simulink model "ex1"  (R2020a)
settings: Solver=VariableStepAuto  StartTime=0.0  StopTime=10.0  RelTol=1e-3

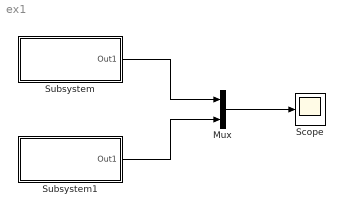
== system ex1 ==
  Mux : Mux  Inputs=2
  Scope : Scope
  Subsystem : Subsystem  mask(subsistem){a1=1, f1=2}
      mask prompts: a1 "a1="; f1 "f1="
      mask help:
      | a1 și f1 reprezintă amplitudinea respectiv frecvența
      | funcției sinus
      mask Help:
      | blocul trasează o funcție sinus de
      | amplitudine a1 și frecvență f1
      mask Callback a1:
      | if str2num(get_param(gcb,'a1'))<0
      |     error('amplitudinea este negativa')
      | end
      mask Callback f1:
      | if str2num(get_param(gcb,'f1'))<0
      |     error('frecventa este negativa')
      | end
  Subsystem1 : Subsystem  mask(subsitem){a2=1, f2=3}
      mask prompts: a2 "a2="; f2 "f2="
      mask help:
      | a1 și f1 reprezintă amplitudinea respectiv frecvența
      | funcției sinus
      mask Help:
      | blocul trasează o funcție sinus de
      | amplitudine a1 și frecvență f1
      mask Callback a2:
      | if str2num(get_param(gcb,'a2'))<0
      |     error('Amplitudinea este negativa!')
      | end
      mask Callback f2:
      | if str2num(get_param(gcb,'f2'))<0
      |     error('Amplitudinea este negativa!')
      | end
  wires:
  Subsystem/1(Out1) -> Mux/1
  Subsystem1/1(Out1) -> Mux/2
  Mux/1 -> Scope/1

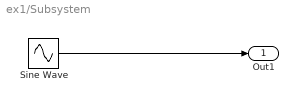
== system ex1/Subsystem ==
  Sine Wave : Sin  Amplitude=a1  Frequency=f1  SampleTime=0
  Out1 : Outport
  wires:
  Sine Wave/1 -> Out1/1

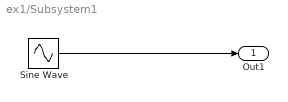
== system ex1/Subsystem1 ==
  Sine Wave : Sin  Amplitude=a2  Frequency=f2  SampleTime=0
  Out1 : Outport
  wires:
  Sine Wave/1 -> Out1/1
